simulink model "eom"  (R2021b)
settings: Solver=ode4  StartTime=0.0  StopTime=100  RelTol=1e-3  EnableMultiTasking=on
PreLoadFcn:
  | PARAMETROS
values from neighbouring files (symbols this model uses):
  b = 0.353    [PARAMETROS.m]    (also in forandtor.m; forandtorPARAM.m)
  CDfront = 0.5    [PARAMETROS.m]    (also in forandtor.m; forandtorPARAM.m)
  CDlat = 0.75    [PARAMETROS.m]    (also in forandtor.m; forandtorPARAM.m)
  CLa = 1    [PARAMETROS.m]    (also in forandtor.m; forandtorPARAM.m)
  CLp = 5    [PARAMETROS.m]    (also in forandtor.m; forandtorPARAM.m)
  CMdeltae = 1    [PARAMETROS.m]    (also in forandtor.m; forandtorPARAM.m)
  CMfq = 1    [PARAMETROS.m]    (also in forandtor.m; forandtorPARAM.m)
  CMw = 10    [PARAMETROS.m]    (also in forandtor.m; forandtorPARAM.m)
  CNdeltar = 1    [PARAMETROS.m]    (also in forandtor.m; forandtorPARAM.m)
  CNfr = 1    [PARAMETROS.m]    (also in forandtor.m; forandtorPARAM.m)
  CNv = 10    [PARAMETROS.m]    (also in forandtor.m; forandtorPARAM.m)
  fullt = 600    [PARAMETROS.m]    (also in forandtor.m; forandtorPARAM.m)
  g = 9.81    [PARAMETROS.m]    (also in eom1.m; eom1PARAM.m)
  Ix = 0.468    [PARAMETROS.m]    (also in eom1.m; eom1PARAM.m)
  Iy = 90.8    [PARAMETROS.m]    (also in eom1.m; eom1PARAM.m)
  Iz = Iy    (= 90.8)    [PARAMETROS.m]    (also in eom1.m; eom1PARAM.m)
  m = 85.3    [PARAMETROS.m]    (also in eom1.m; eom1PARAM.m)
  Sfront = 0.0127    [PARAMETROS.m]    (also in forandtor.m; forandtorPARAM.m)
  Slat = 1.2049    [PARAMETROS.m]    (also in forandtor.m; forandtorPARAM.m)
  Sstab = 0.45    [PARAMETROS.m]    (also in forandtor.m; forandtorPARAM.m)
  Swing = 0.4525    [PARAMETROS.m]    (also in forandtor.m; forandtorPARAM.m)
libraries: aerolibanim x6, aerolibatmos2 x3
(part 2 of 2)

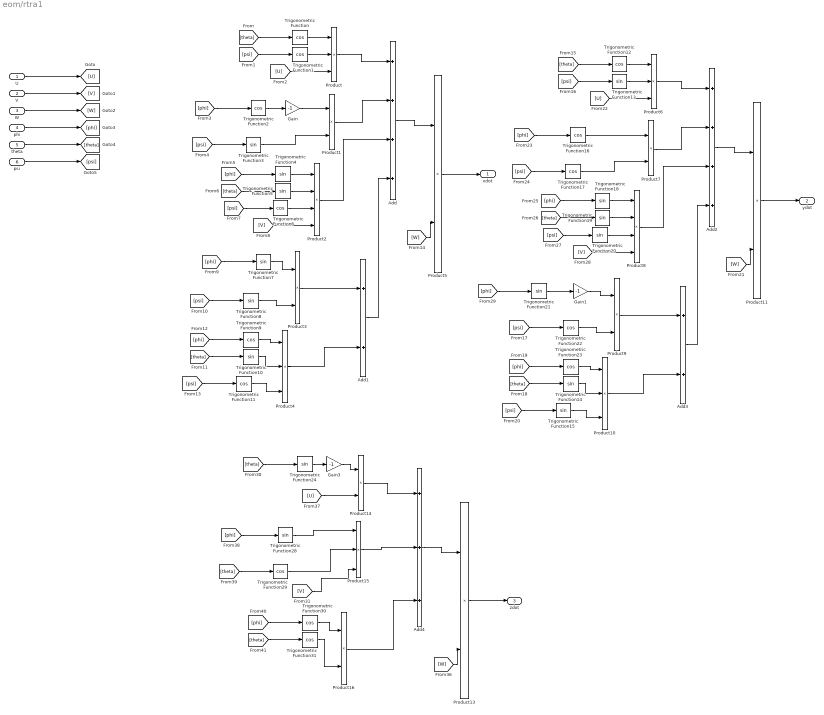
== system eom/rtra1 ==
  U : Inport
  V : Inport  Port=2
  W : Inport  Port=3
  phi : Inport  Port=4
  theta : Inport  Port=5
  psi : Inport  Port=6
  Add : Sum  Inputs=++++
  Add1 : Sum
  Add2 : Sum  Inputs=++++
  Add3 : Sum
  Add4 : Sum  Inputs=+++
  Gain : Gain  Gain=-1
  Gain1 : Gain  Gain=-1
  Gain3 : Gain  Gain=-1
  Product{,4,6,10,15} (5 alike) : Product  Inputs=3
  Product{1,3,5,7,9,11,13..14,16} (9 alike) : Product
  Product2 : Product  Inputs=4
  Product8 : Product  Inputs=4
  Trigonometric Function{,1..2,6,9,11..12,16..17,22..23,29..31} (14 alike) : Trigonometry  Operator=cos
  Trigonometric Function{3..5,7..8,10,13..15,18..21,24,28} (15 alike) : Trigonometry
  xdot : Outport
  ydot : Outport  Port=2
  zdot : Outport  Port=3
  wires:
  U/1 -> [U]
  V/1 -> [V]
  W/1 -> [W]
  phi/1 -> [phi]
  theta/1 -> [theta]
  psi/1 -> [psi]
  [theta] -> Trigonometric Function/1
  Trigonometric Function/1 -> Product/1
  [psi] -> Trigonometric Function1/1
  Trigonometric Function1/1 -> Product/2
  [U] -> Product/3
  Product/1 -> Add/1
  [phi] -> Trigonometric Function2/1
  Trigonometric Function2/1 -> Gain/1
  [psi] -> Trigonometric Function3/1
  Gain/1 -> Product1/1
  Trigonometric Function3/1 -> Product1/2
  Product1/1 -> Add/2
  [theta] -> Trigonometric Function5/1
  Trigonometric Function5/1 -> Product2/2
  [phi] -> Trigonometric Function4/1
  Trigonometric Function4/1 -> Product2/1
  [V] -> Product2/4
  Product2/1 -> Add/3
  [psi] -> Trigonometric Function6/1
  Trigonometric Function6/1 -> Product2/3
  [psi] -> Trigonometric Function8/1
  Trigonometric Function7/1 -> Product3/1
  Trigonometric Function8/1 -> Product3/2
  [phi] -> Trigonometric Function7/1
  Trigonometric Function10/1 -> Product4/2
  Trigonometric Function9/1 -> Product4/1
  [theta] -> Trigonometric Function10/1
  [phi] -> Trigonometric Function9/1
  Add1/1 -> Add/4
  Product3/1 -> Add1/1
  Product4/1 -> Add1/2
  Trigonometric Function11/1 -> Product4/3
  [psi] -> Trigonometric Function11/1
  [W] -> Product5/2
  Add/1 -> Product5/1
  Product5/1 -> xdot/1
  [psi] -> Trigonometric Function13/1
  Trigonometric Function16/1 -> Product7/1
  [V] -> Product8/4
  Trigonometric Function13/1 -> Product6/2
  [psi] -> Trigonometric Function20/1
  [psi] -> Trigonometric Function17/1
  Add2/1 -> Product11/1
  Trigonometric Function20/1 -> Product8/3
  Trigonometric Function18/1 -> Product8/1
  [theta] -> Trigonometric Function19/1
  Product8/1 -> Add2/3
  Trigonometric Function17/1 -> Product7/2
  Trigonometric Function21/1 -> Gain1/1
  Product10/1 -> Add3/2
  [phi] -> Trigonometric Function23/1
  [theta] -> Trigonometric Function12/1
  [theta] -> Trigonometric Function14/1
  Trigonometric Function23/1 -> Product10/1
  Trigonometric Function14/1 -> Product10/2
  Product6/1 -> Add2/1
  Product11/1 -> ydot/1
  [psi] -> Trigonometric Function15/1
  Product9/1 -> Add3/1
  Trigonometric Function15/1 -> Product10/3
  [W] -> Product11/2
  Trigonometric Function22/1 -> Product9/2
  [phi] -> Trigonometric Function16/1
  [phi] -> Trigonometric Function21/1
  Product7/1 -> Add2/2
  Add3/1 -> Add2/4
  Trigonometric Function12/1 -> Product6/1
  Trigonometric Function19/1 -> Product8/2
  [phi] -> Trigonometric Function18/1
  [U] -> Product6/3
  [psi] -> Trigonometric Function22/1
  Gain1/1 -> Product9/1
  Trigonometric Function31/1 -> Product16/2
  [phi] -> Trigonometric Function28/1
  [W] -> Product13/2
  Product14/1 -> Add4/1
  Trigonometric Function28/1 -> Product15/1
  [theta] -> Trigonometric Function24/1
  Product13/1 -> zdot/1
  Product15/1 -> Add4/2
  Trigonometric Function29/1 -> Product15/2
  Product16/1 -> Add4/3
  Trigonometric Function30/1 -> Product16/1
  [theta] -> Trigonometric Function31/1
  Add4/1 -> Product13/1
  [theta] -> Trigonometric Function29/1
  [phi] -> Trigonometric Function30/1
  Trigonometric Function24/1 -> Gain3/1
  Gain3/1 -> Product14/1
  [U] -> Product14/2
  [V] -> Product15/3

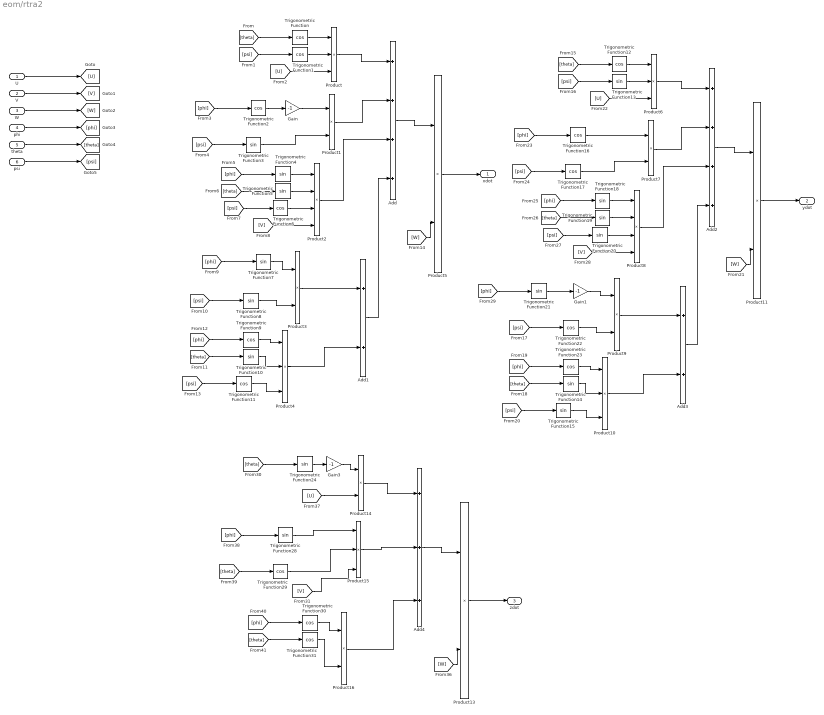
== system eom/rtra2 ==
  U : Inport
  V : Inport  Port=2
  W : Inport  Port=3
  phi : Inport  Port=4
  theta : Inport  Port=5
  psi : Inport  Port=6
  Add : Sum  Inputs=++++
  Add1 : Sum
  Add2 : Sum  Inputs=++++
  Add3 : Sum
  Add4 : Sum  Inputs=+++
  Gain : Gain  Gain=-1
  Gain1 : Gain  Gain=-1
  Gain3 : Gain  Gain=-1
  Product{,4,6,10,15} (5 alike) : Product  Inputs=3
  Product{1,3,5,7,9,11,13..14,16} (9 alike) : Product
  Product2 : Product  Inputs=4
  Product8 : Product  Inputs=4
  Trigonometric Function{,1..2,6,9,11..12,16..17,22..23,29..31} (14 alike) : Trigonometry  Operator=cos
  Trigonometric Function{3..5,7..8,10,13..15,18..21,24,28} (15 alike) : Trigonometry
  xdot : Outport
  ydot : Outport  Port=2
  zdot : Outport  Port=3
  wires:
  U/1 -> [U]
  V/1 -> [V]
  W/1 -> [W]
  phi/1 -> [phi]
  theta/1 -> [theta]
  psi/1 -> [psi]
  [theta] -> Trigonometric Function/1
  Trigonometric Function/1 -> Product/1
  [psi] -> Trigonometric Function1/1
  Trigonometric Function1/1 -> Product/2
  [U] -> Product/3
  Product/1 -> Add/1
  [phi] -> Trigonometric Function2/1
  Trigonometric Function2/1 -> Gain/1
  [psi] -> Trigonometric Function3/1
  Gain/1 -> Product1/1
  Trigonometric Function3/1 -> Product1/2
  Product1/1 -> Add/2
  [theta] -> Trigonometric Function5/1
  Trigonometric Function5/1 -> Product2/2
  [phi] -> Trigonometric Function4/1
  Trigonometric Function4/1 -> Product2/1
  [V] -> Product2/4
  Product2/1 -> Add/3
  [psi] -> Trigonometric Function6/1
  Trigonometric Function6/1 -> Product2/3
  [psi] -> Trigonometric Function8/1
  Trigonometric Function7/1 -> Product3/1
  Trigonometric Function8/1 -> Product3/2
  [phi] -> Trigonometric Function7/1
  Trigonometric Function10/1 -> Product4/2
  Trigonometric Function9/1 -> Product4/1
  [theta] -> Trigonometric Function10/1
  [phi] -> Trigonometric Function9/1
  Add1/1 -> Add/4
  Product3/1 -> Add1/1
  Product4/1 -> Add1/2
  Trigonometric Function11/1 -> Product4/3
  [psi] -> Trigonometric Function11/1
  [W] -> Product5/2
  Add/1 -> Product5/1
  Product5/1 -> xdot/1
  [psi] -> Trigonometric Function13/1
  Trigonometric Function16/1 -> Product7/1
  [V] -> Product8/4
  Trigonometric Function13/1 -> Product6/2
  [psi] -> Trigonometric Function20/1
  [psi] -> Trigonometric Function17/1
  Add2/1 -> Product11/1
  Trigonometric Function20/1 -> Product8/3
  Trigonometric Function18/1 -> Product8/1
  [theta] -> Trigonometric Function19/1
  Product8/1 -> Add2/3
  Trigonometric Function17/1 -> Product7/2
  Trigonometric Function21/1 -> Gain1/1
  Product10/1 -> Add3/2
  [phi] -> Trigonometric Function23/1
  [theta] -> Trigonometric Function12/1
  [theta] -> Trigonometric Function14/1
  Trigonometric Function23/1 -> Product10/1
  Trigonometric Function14/1 -> Product10/2
  Product6/1 -> Add2/1
  Product11/1 -> ydot/1
  [psi] -> Trigonometric Function15/1
  Product9/1 -> Add3/1
  Trigonometric Function15/1 -> Product10/3
  [W] -> Product11/2
  Trigonometric Function22/1 -> Product9/2
  [phi] -> Trigonometric Function16/1
  [phi] -> Trigonometric Function21/1
  Product7/1 -> Add2/2
  Add3/1 -> Add2/4
  Trigonometric Function12/1 -> Product6/1
  Trigonometric Function19/1 -> Product8/2
  [phi] -> Trigonometric Function18/1
  [U] -> Product6/3
  [psi] -> Trigonometric Function22/1
  Gain1/1 -> Product9/1
  Trigonometric Function31/1 -> Product16/2
  [phi] -> Trigonometric Function28/1
  [W] -> Product13/2
  Product14/1 -> Add4/1
  Trigonometric Function28/1 -> Product15/1
  [theta] -> Trigonometric Function24/1
  Product13/1 -> zdot/1
  Product15/1 -> Add4/2
  Trigonometric Function29/1 -> Product15/2
  Product16/1 -> Add4/3
  Trigonometric Function30/1 -> Product16/1
  [theta] -> Trigonometric Function31/1
  Add4/1 -> Product13/1
  [theta] -> Trigonometric Function29/1
  [phi] -> Trigonometric Function30/1
  Trigonometric Function24/1 -> Gain3/1
  Gain3/1 -> Product14/1
  [U] -> Product14/2
  [V] -> Product15/3
